simulink model "c6problem1simulation"  (R2023b)
settings: Solver=VariableStepAuto  StartTime=0.0  StopTime=30  RelTol=1e-10
values from neighbouring files (symbols this model uses):
  d0 = 0    [c6problem1.m]
  d1 = 1    [c6problem1.m]
  d2 = 5    [c6problem1.m]
  den1 = [1 3 2 0]    [c6problem1.m]
  den2 = [2 1]    [c6problem1.m]
  eps0 = 0    [c6problem1.m]
  eps1 = 0    [c6problem1.m]
  eps2 = 1    [c6problem1.m]
  num1 = 10    [c6problem1.m]
  num2 = 3    [c6problem1.m]
settings Model: Creator=klysm  LastModifiedBy=klysm

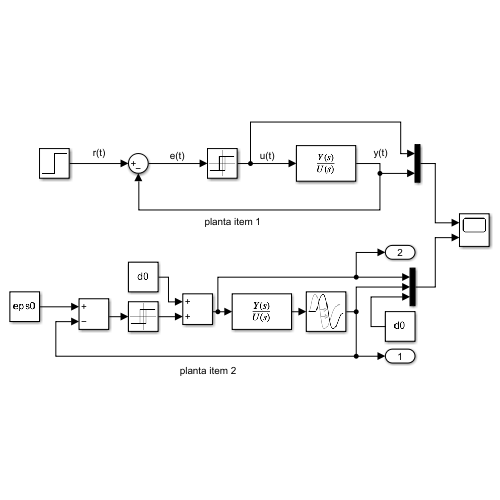
[thumbnail: Simulink's stored preview of the top-level diagram]
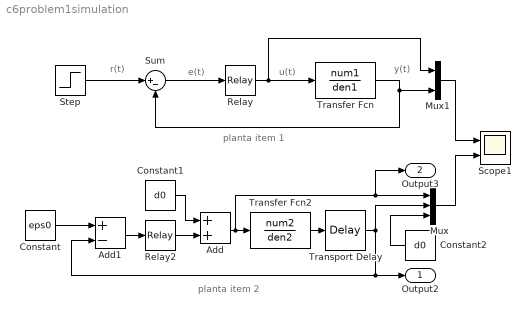
== system c6problem1simulation ==
  note: planta item 1
  note: e(t)
  note: u(t)
  note: y(t)
  note: r(t)
  note: planta item 2
  Add : Sum
  Add1 : Sum  Inputs=+-
  Constant : Constant  Value=eps0
  Constant1 : Constant  Value=d0
  Constant2 : Constant  Value=d0
  Mux : Mux  Inputs=3
  Mux1 : Mux  Inputs=2
  Relay : Relay  OnSwitchValue=eps1  OffSwitchValue=eps1  OnOutputValue=d1  OffOutputValue=-d1
  Relay2 : Relay  OnSwitchValue=eps2  OffSwitchValue=eps2  OnOutputValue=d2  OffOutputValue=-d2
  Scope1 : Scope  NumInputPorts=2
  Step : Step  Before=-1  SampleTime=1
  Sum : Sum  Inputs=|+-
  Transfer Fcn : TransferFcn  Numerator=num1  Denominator=den1
  Transfer Fcn2 : TransferFcn  Numerator=num2  Denominator=den2
  Transport Delay : TransportDelay  DelayTime=0.1
  Output2 : Outport
  Output3 : Outport  Port=2
  wires:
  Transfer Fcn/1 -> Mux1/2, Sum/2
  Relay2/1 -> Add/2
  Add1/1 -> Relay2/1
  Constant1/1 -> Add/1
  Constant/1 -> Add1/1
  Add/1 -> Output3/1, Mux/1, Transfer Fcn2/1
  Transfer Fcn2/1 -> Transport Delay/1
  Mux/1 -> Scope1/2
  Constant2/1 -> Mux/3
  Transport Delay/1 -> Add1/2, Output2/1, Mux/2
  Mux1/1 -> Scope1/1
  Step/1 -> Sum/1
  Sum/1 -> Relay/1
  Relay/1 -> Mux1/1, Transfer Fcn/1
